simulink model "car_model_FIXED"  (R2022b)
settings: Solver=VariableStepAuto  StartTime=0.0  StopTime=60  RelTol=1e-3
values from neighbouring files (symbols this model uses):
  ABS_MAX_TORQUE = [25 25 25 25]    [workspace.mat]
  ABS_MAX_TRQ_CMD = 50    [workspace.mat]
  ABS_MIN_TORQUE = [0.01 0.01 0.01 0.01]    [workspace.mat]
  acc_IC = 0    [workspace.mat]
  ACCELERATION_MAX = 30    [workspace.mat]
  ActSuspDutyCycle = 1    [workspace.mat]
  Aeq_left = [0.305756190204 0.308857786592 0.311945941182 0.315020811431 0.318082554689 0.321131328186 0.324167289011 0.327190594103 0.330201400225 0.333199863958 0.336186141681 0.339160389558 ... (261 elements, 1x261)]    [workspace.mat]
  Aeq_right = [-0.961664782545 -0.959835898365 -0.957982924115 -0.956106413788 -0.954206913862 -0.952284963337 -0.950341093764 -0.948375829284 -0.946389686656 -0.944383175301 -0.942356797333 -0.940311047601 ... (261 elements, 1x261)]    [workspace.mat]
  alpha_error = 0.1    [workspace.mat]
  ang_acc_hystersesis = 0.1    [workspace.mat]
  ang_IC = 0    [workspace.mat]
  ang_vel_IC = 0    [workspace.mat]
  area_air = 0.15    [workspace.mat]
  axb = -5    [workspace.mat]
  battery_current_IC = 0    [workspace.mat]
  BATTERY_CURRENT_MAX = 140    [workspace.mat]
  BATTERY_CURRENT_MIN = 0    [workspace.mat]
  battery_FT_IC = 300    [workspace.mat]
  battery_T_IC = 300    [workspace.mat]
  BATTERY_TEMPERATURE_MAX = 60    [workspace.mat]
  BATTERY_TEMPERATURE_MIN = 0    [workspace.mat]
  battery_voltage_IC = 332    [workspace.mat]
  BATTERY_VOLTAGE_MAX = 340    [workspace.mat]
  BATTERY_VOLTAGE_MIN = 60    [workspace.mat]
  br = 0.01    [workspace.mat]
  brake_bias = [0.35 0.35 0.15 0.15]    [workspace.mat]
  Brake_Pressure_IC = 1    [workspace.mat]
  ccl_IC = 0    [workspace.mat]
  CENTER_STEER_ANGLE_MAX = 130    [workspace.mat]
  covarience_matrix_IC = [0.001 0 0 0 0 0 0 0 0 0 0 0 ... (784 elements, 28x28)]    [workspace.mat]
  CURRENT_BUFFER = 25    [workspace.mat]
  cy_sweep = [13568.4166816 14020.2069783 14456.754831 14879.7402576 15289.7264712 15687.2766846 16072.954111 16447.3219632 16810.9434544 17164.3817975 17508.2002054 17842.9618912 ... (101 elements, 1x101)]    [workspace.mat]
  dB = 0.001    [workspace.mat]
  dcl_IC = 140    [workspace.mat]
  DCL_MAX = 130    [workspace.mat]
  DCL_MIN = 0    [workspace.mat]
  deadband_angle = 12    [workspace.mat]
  dIndex = 50    [workspace.mat]
  driver_t = 0.015    [workspace.mat]
  dt_OFF = 4.5    [workspace.mat]
  dt_ON = 7.5    [workspace.mat]
  dTx = 0.01    [workspace.mat]
  dx = 0.1    [workspace.mat]
  dZ = 0.295    [workspace.mat]
  efficiency_grid = [0.759500051293 0.787587791453 0.809832189108 0.826747821898 0.837164543102 0.842744381136 0.842258400104 0.838611650621 0.82826195101 0.814029316176 0.795690627225 0.7759791486 ... (2782 elements, 26x107)]    [workspace.mat]
  F0z = [0 0]    [workspace.mat]
  forward_look_straight = 5    [workspace.mat]
  forward_look_turn = 15    [workspace.mat]
  Fz_IC = 539.55    [workspace.mat]
  Fz_sweep = [200 210 220 230 240 250 260 270 280 290 300 310 ... (101 elements, 1x101)]    [workspace.mat]
  g = 9.81    [workspace.mat]
  GAIN_ABS = 100    [workspace.mat]
  gearbox_efficiency = [0.8 0.8 0.8 0.8]    [workspace.mat]
  gps_counter_IC = 0    [workspace.mat]
  gps_hz = 0.01    [workspace.mat]
  gr = [8.74786324786 8.74786324786 8.74786324786 8.74786324786]    [workspace.mat]
  I = 0    [workspace.mat]
  I_Driver = 1    [workspace.mat]
  indicies = [3 3.5 4 0.5 1 1.5 2 2.5 3 3.5 4 0.5 ... (27 elements, 1x27)]    [workspace.mat]
  IYY = 0.3    [workspace.mat]
  kx_sweep = [8779.958 9178.302 9576.646 9974.99 10373.334 10771.678 11170.022 11568.366 11966.71 12365.054 12763.398 13161.742 ... (101 elements, 1x101)]    [workspace.mat]
  l = [0.772 0.772]    [workspace.mat]
  lambda_star = 0.15    [workspace.mat]
  low_V_SA = 0.001    [workspace.mat]
  lr = 35    [workspace.mat]
  m_all = 220    [workspace.mat]
  m_body = 180    [workspace.mat]
  m_unsprung = [6 6 14 14]    [workspace.mat]
  MAG_MAX = 200    [workspace.mat]
  Max_Brake_Pressure = 100000000    [workspace.mat]
  Max_Driver_Input = 1    [workspace.mat]
  MAX_DTHETA_DRIVER = 360    [workspace.mat]
  MAX_I_Driver = 1    [workspace.mat]
  MAX_STEERING_ADJUST = 15    [workspace.mat]
  max_yaw = [0.705271610162 0.928228152446 1.12280857731 1.14131008363 1.08727026041 1.01377803859 0.938114723816 0.8718206875 0.815009168116 0.767481919497 0.727119764215 0.694403589394 ... (15 elements, 1x15)]    [workspace.mat]
  Min_Brake_Pressure = 1    [workspace.mat]
  Min_Driver_Input = 0    [workspace.mat]
  min_velocity_regen = 1.4    [workspace.mat]
  motor_current_IC = 0    [workspace.mat]
  MOTOR_CURRENT_MAX = 70    [workspace.mat]
  MOTOR_CURRENT_MIN = 0    [workspace.mat]
  MOTOR_ENABLE = [0 0 1 1]    [workspace.mat]
  motor_FT_IC = 300    [workspace.mat]
  motor_T_IC = 300    [workspace.mat]
  MOTOR_TEMPERATURE_MAX = 100    [workspace.mat]
  MOTOR_TEMPERATURE_MIN = 0    [workspace.mat]
  motor_voltage_IC = 332    [workspace.mat]
  MOTOR_VOLTAGE_MAX = 340    [workspace.mat]
  MOTOR_VOLTAGE_MIN = 90    [workspace.mat]
  motorControllerCurve = [25  260; 50  130; 75  0]    [workspace.mat]
  motorTempCurve = [140 138.6 134.4 127.4 117.6 105 89.6 71.4 50.4 26.6 0]    [workspace.mat]
  motorTempX = [75 77 79 81 83 85 87 89 91 93 95]    [workspace.mat]
  mu_star = 0.5    [workspace.mat]
  mx_sweep = [3.38348 3.3655067 3.3477908 3.3303323 3.3131312 3.2961875 3.2795012 3.2630723 3.2469008 3.2309867 3.21533 3.1999307 ... (101 elements, 1x101)]    [workspace.mat]
  my_sweep = [3.036232 3.015241699 2.994987032 2.975452753 2.956623616 2.938484375 2.921019784 2.904214597 2.888053568 2.872521451 2.857603 2.843282969 ... (101 elements, 1x101)]    [workspace.mat]
  noise_state = [1e-06 1e-06 1e-06 1e-06 0.005 0.005 0.005 1e-06 1e-06 1e-06 1e-06 1e-06 ... (28 elements, 28x1)]    [workspace.mat]
  omega_IC = 0    [workspace.mat]
  OMEGA_MAX = 150    [workspace.mat]
  OMEGA_MIN = 0    [workspace.mat]
  ORIENTATION_MAX = 360    [workspace.mat]
  P = 2    [workspace.mat]
  P_Driver = 0.7    [workspace.mat]
  P_High_Speed = 0.1    [workspace.mat]
  P_Steering_Adjust = 2    [workspace.mat]
  P_Straight_Adjust = 5    [workspace.mat]
  pos_IC = 0    [workspace.mat]
  POS_MAX = 300    [workspace.mat]
  q_thresh = 0.3    [workspace.mat]
  RE = 0.223    [workspace.mat]
  rho = 1.225    [workspace.mat]
  s = [0.649 0.621]    [workspace.mat]
  selected_maxvm = [49.86390724 16.21289794 8.219813569 8.05215527 7.103352929 8.35634983 13.87515039 8.72402841 22.75224945 36.67909339 19.32001297 25.09036962 ... (63 elements, 21x3)]    [workspace.mat]
  selected_sweep = [3 3 3 3 3 3 3 3 3 3 3 3 ... (1288 elements, 644x2)]    [workspace.mat]
  selected_track = [inf inf inf inf inf inf inf inf inf inf inf inf ... (37971 elements, 4219x9)]    [workspace.mat]
  shock_length_IC = 0.1    [workspace.mat]
  SHOCK_LENGTH_MAX = 0.25    [workspace.mat]
  SHOCK_LENGTH_MIN = 0    [workspace.mat]
  state_IC = [1 0 0 0 0 0 0 0 0 0 0 0 ... (28 elements, 28x1)]    [workspace.mat]
  steering_sweep = [0 5 10 15 20 25 30 35 40 45 50 55 ... (27 elements, 1x27)]    [workspace.mat]
  steering_Up_Grid = [0.551231966244 8.36038106007 16.1333806643 23.9559539118 31.8240691982 39.7561724339 47.7157531433 55.7845698794 64.1341708168 73.0798046026 82.7903081349 93.1297322155 ... (615 elements, 41x15)]    [workspace.mat]
  ... (+25 more)
undefined symbols (not defined in the file or in its folder): ax, ay, az, covA, covG, covM, covP, covV, DiscIntNeverNeededParam, fusion_t, fusion_t_sim, gps_ratio, IMU_accel, IMU_gyro, imu_hz, IMU_mag, location_lla_IC, p, phi, psi, q, r, sus, theta, trn, veh, VEH, whl, X, Xdot, Y, Ydot, Z, Zdot
libraries: fl_lib x82, nesl_utility x32, vehdynlibtire x10, vehdynlibsuspension x8, simulink x5, autolibutils x5, sharedtransform x5, sdl_lib x4, EngineCoolingComponents_lib x4, slpidlib x3, SimscapeFluids_lib x3, shared6dof x2
(part 3 of 14)

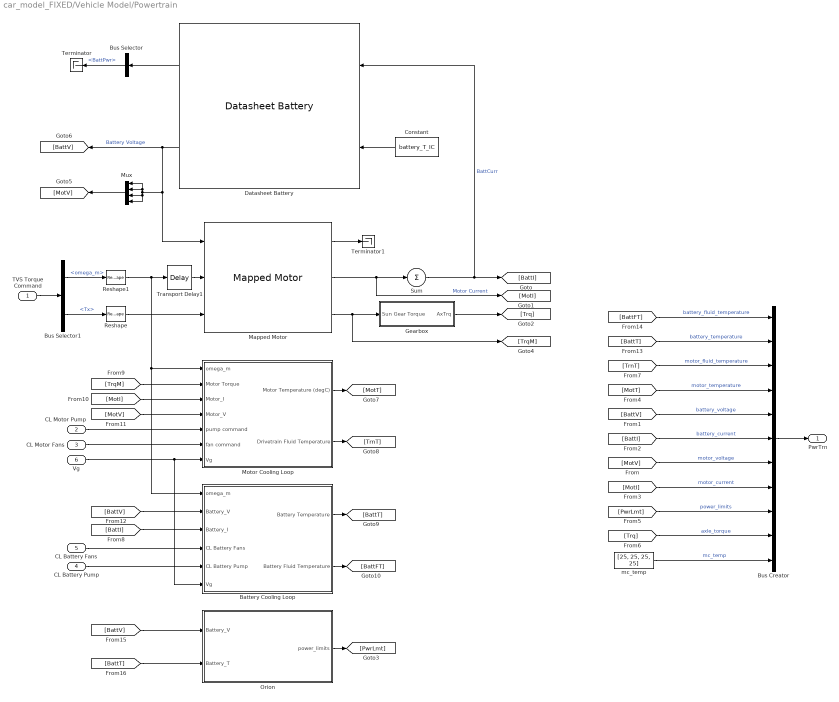
== system car_model_FIXED/Vehicle Model/Powertrain ==
  TVS Torque Command : Inport
  CL Motor Pump : Inport  Port=2
  CL Motor Fans : Inport  Port=3
  CL Battery Pump : Inport  Port=4
  CL Battery Fans : Inport  Port=5
  Vg : Inport  Port=6
  Battery Cooling Loop : Subsystem
  Bus Creator : BusCreator  Inputs=11
  Bus Selector : BusSelector  OutputSignals=BattPwr
  Bus Selector1 : BusSelector  OutputSignals=omega_m,Tx
  Constant : Constant  Value=battery_T_IC
  Datasheet Battery : autolibdatasheetbattery/Datasheet Battery  CapacityCtrl=Parameter  OutputVlt=Filtered  BattChargeMax=BattCap  Em=Em  CapLUTBp=SOC  RInt=RESISTANCE  BattTempBp=TEMPERATURE  CapSOCBp=SOC  Ns=Ns  Np=Np  BattCapInit=BattCap_I  Tc=Battery_tau  Vinit=battery_voltage_IC  RefBlkName='autolibdatasheetbattery/Datasheet Battery'
  Gearbox : Subsystem
  Mapped Motor : autolibmappedmotor/Mapped Motor  port_config=Speed  param_by=Tabulated torque-speed envelope  w_t=rpm_sweep  T_t=max_torque_grid(end,:)  torque_max=.1  power_max=30  Tc=Motor_tau  param_loss=Tabulated efficiency data  eff=100  w_eff=375  T_eff=0.08  Piron=0  Pbase=0  w_eff_bp=rpm_sweep  T_eff_bp=torque_sweep  Temp_eff_bp=[233.15 293.15 373.15]  losses_table=[1.49 1.67 2.21 3.10; 0.42 0.69 1.14 2.03; 0.06 0.24 0.78 1.68; 0.42 0.69 1.14 2.03; 1.49 1.67 2.21 3.10]  losses_table_3d=cat(3,[1.49 1.67 2.21 3.10; 0.42 0.69 1.14 2.03; 0.06 0.24 0.78 1.68; 0.42 0.69 1.14 2.03; 1.49 1.67 2.21 3.10],[1.49 1.67 2.21 3.10; 0.42 0.69 1.14 2.03; 0.06 0.24 0.78 1.68; 0.42 0.69 1.14 2.03; 1.49 1.67 2.21 3.10],[1.49 1.67 2.21 3.10; 0.42 0.69 1.14 2.03; 0.06 0.24 0.78 1.68; 0.42 0.69 1.14 2.03; 1.49 1.67 2.21 3.10])  efficiency_table=100*efficiency_grid'  efficiency_table_3d=cat(3,[95 95 95 95; 95 95 95 95; 95 95 95 95; 95 95 95 95; 95 95 95 95],[95 95 95 95; 95 95 95 95; 95 95 95 95; 95 95 95 95; 95 95 95 95],[95 95 95 95; 95 95 95 95; 95 95 95 95; 95 95 95 95; 95 95 95 95])  J=5e-6  b=1e-5  omega_o=0  T_t_extended=[1.32786372122435 1.93296548257099 2.5425618526431 3.15736795662177 3.77818881981173 4.40971488438617 5.05604488344693 5.69719862521611 6.35896558084689 7.05699514881516 7.75957227021141 8.48856911751552 9.2939724316526 10.1031648805232 10.9920408781878 11.9746245835295 13.0147067052248 14.1174245714548 15.288285754278 16.5327710759749 17.9226945866055 19.3096243918455 20.7636741817153 22.2031334917467 23.663316115528 25 25 25 25 25 25 25 25 25 25 25 25 25 25 25 25 25 25 25 25 25 25 25 25 25 25 25 25 25 25 25 25 25 25 25 25 25 25 25 25 25 25 25 25 25 25 25 25 25 25 25 25 25 25 25 25 25 25 25 25 25 25 25 25 25 25 25 25 25 25 25 25 25 25 25 25 25 25 25 25 25 25 25 25 25 25 25 25 25 25 25 25 25 25 25 25 25 25 25 25 25 25 25 25 25 25 25 25 25 25 25 25 25 25 25 25 25 25 25 25 25 25 25 25 25 25 25 25 25 25 25 25 25 25 25 25 25 25 25 25 25 25 25 25 25 25 25 25 25 25 25 25 25 25 25 25 25 25 25 25 25 25 25 23.663316115528 22.2031334917467 20.7636741817153 19.3096243918455 17.9226945866055 16.5327710759749 15.288285754278 14.1174245714548 13.0147067052248 11.9746245835295 10.9920408781878 10.1031648805232 9.2939724316526 8.48856911751552 7.75957227021141 7.05699514881516 6.35896558084689 5.69719862521611 5.05604488344693 4.40971488438617 3.77818881981173 3.15736795662177 2.5425618526431 1.93296548257099 1.32786372122435]  w_t_extended=[-1100 -1089.62264150943 -1079.24528301887 -1068.8679245283 -1058.49056603774 -1048.11320754717 -1037.7358490566 -1027.35849056604 -1016.98113207547 -1006.60377358491 -996.22641509434 -985.849056603774 -975.471698113208 -965.094339622642 -954.716981132075 -944.339622641509 -933.962264150943 -923.584905660377 -913.207547169811 -902.830188679245 -892.452830188679 -882.075471698113 -871.698113207547 -861.320754716981 -850.943396226415 -840.566037735849 -830.188679245283 -819.811320754717 -809.433962264151 -799.056603773585 -788.679245283019 -778.301886792453 -767.924528301887 -757.547169811321 -747.169811320755 -736.792452830189 -726.415094339623 -716.037735849057 -705.660377358491 -695.283018867925 -684.905660377358 -674.528301886792 -664.150943396226 -653.77358490566 -643.396226415094 -633.018867924528 -622.641509433962 -612.264150943396 -601.88679245283 -591.509433962264 -581.132075471698 -570.754716981132 -560.377358490566 -550 -539.622641509434 -529.245283018868 -518.867924528302 -508.490566037736 -498.11320754717 -487.735849056604 -477.358490566038 -466.981132075472 -456.603773584906 -446.22641509434 -435.849056603774 -425.471698113208 -415.094339622641 -404.716981132075 -394.339622641509 -383.962264150943 -373.584905660377 -363.207547169811 -352.830188679245 -342.452830188679 -332.075471698113 -321.698113207547 -311.320754716981 -300.943396226415 -290.566037735849 -280.188679245283 -269.811320754717 -259.433962264151 -249.056603773585 -238.679245283019 -228.301886792453 -217.924528301887 -207.547169811321 -197.169811320755 -186.792452830189 -176.415094339623 -166.037735849057 -155.660377358491 -145.283018867925 -134.905660377358 -124.528301886792 -114.150943396226 -103.77358490566 -93.3962264150943 -83.0188679245283 -72.6415094339623 -62.2641509433962 -51.8867924528302 -41.5094339622642 -31.1320754716981 -20.7547169811321 -10.377358490566 0 10.377358490566 20.7547169811321 31.1320754716981 41.5094339622642 51.8867924528302 62.2641509433962 72.6415094339623 83.0188679245283 93.3962264150943 103.77358490566 114.150943396226 124.528301886792 134.905660377358 145.283018867925 155.660377358491 166.037735849057 176.415094339623 186.792452830189 197.169811320755 207.547169811321 217.924528301887 228.301886792453 238.679245283019 249.056603773585 259.433962264151 269.811320754717 280.188679245283 290.566037735849 300.943396226415 311.320754716981 321.698113207547 332.075471698113 342.452830188679 352.830188679245 363.207547169811 373.584905660377 383.962264150943 394.339622641509 404.716981132075 415.094339622641 425.471698113208 435.849056603774 446.22641509434 456.603773584906 466.981132075472 477.358490566038 487.735849056604 498.11320754717 508.490566037736 518.867924528302 529.245283018868 539.622641509434 550 560.377358490566 570.754716981132 581.132075471698 591.509433962264 601.88679245283 612.264150943396 622.641509433962 633.018867924528 643.396226415094 653.77358490566 664.150943396226 674.528301886792 684.905660377358 695.283018867925 705.660377358491 716.037735849057 726.415094339623 736.792452830189 747.169811320755 757.547169811321 767.924528301887 778.301886792453 788.679245283019 799.056603773585 809.433962264151 819.811320754717 830.188679245283 840.566037735849 850.943396226415 861.320754716981 871.698113207547 882.075471698113 892.452830188679 902.830188679245 913.207547169811 923.584905660377 933.962264150943 944.339622641509 954.716981132075 965.094339622642 975.471698113208 985.849056603774 996.22641509434 1006.60377358491 1016.98113207547 1027.35849056604 1037.7358490566 1048.11320754717 1058.49056603774 1068.8679245283 1079.24528301887 1089.62264150943 1100]  KLossIron=0  KLossCopper=0  x_w_eff_vec=[-1100 -1089.62264150943 -1079.24528301887 -1068.8679245283 -1058.49056603774 -1048.11320754717 -1037.7358490566 -1027.35849056604 -1016.98113207547 -1006.60377358491 -996.22641509434 -985.849056603774 -975.471698113208 -965.094339622642 -954.716981132075 -944.339622641509 -933.962264150943 -923.584905660377 -913.207547169811 -902.830188679245 -892.452830188679 -882.075471698113 -871.698113207547 -861.320754716981 -850.943396226415 -840.566037735849 -830.188679245283 -819.811320754717 -809.433962264151 -799.056603773585 -788.679245283019 -778.301886792453 -767.924528301887 -757.547169811321 -747.169811320755 -736.792452830189 -726.415094339623 -716.037735849057 -705.660377358491 -695.283018867925 -684.905660377358 -674.528301886792 -664.150943396226 -653.77358490566 -643.396226415094 -633.018867924528 -622.641509433962 -612.264150943396 -601.88679245283 -591.509433962264 -581.132075471698 -570.754716981132 -560.377358490566 -550 -539.622641509434 -529.245283018868 -518.867924528302 -508.490566037736 -498.11320754717 -487.735849056604 -477.358490566038 -466.981132075472 -456.603773584906 -446.22641509434 -435.849056603774 -425.471698113208 -415.094339622641 -404.716981132075 -394.339622641509 -383.962264150943 -373.584905660377 -363.207547169811 -352.830188679245 -342.452830188679 -332.075471698113 -321.698113207547 -311.320754716981 -300.943396226415 -290.566037735849 -280.188679245283 -269.811320754717 -259.433962264151 -249.056603773585 -238.679245283019 -228.301886792453 -217.924528301887 -207.547169811321 -197.169811320755 -186.792452830189 -176.415094339623 -166.037735849057 -155.660377358491 -145.283018867925 -134.905660377358 -124.528301886792 -114.150943396226 -103.77358490566 -93.3962264150943 -83.0188679245283 -72.6415094339623 -62.2641509433962 -51.8867924528302 -41.5094339622642 -31.1320754716981 -20.7547169811321 -10.377358490566 0 10.377358490566 20.7547169811321 31.1320754716981 41.5094339622642 51.8867924528302 62.2641509433962 72.6415094339623 83.0188679245283 93.3962264150943 103.77358490566 114.150943396226 124.528301886792 134.905660377358 145.283018867925 155.660377358491 166.037735849057 176.415094339623 186.792452830189 197.169811320755 207.547169811321 217.924528301887 228.301886792453 238.679245283019 249.056603773585 259.433962264151 269.811320754717 280.188679245283 290.566037735849 300.943396226415 311.320754716981 321.698113207547 332.075471698113 342.452830188679 352.830188679245 363.207547169811 373.584905660377 383.962264150943 394.339622641509 404.716981132075 415.094339622641 425.471698113208 435.849056603774 446.22641509434 456.603773584906 466.981132075472 477.358490566038 487.735849056604 498.11320754717 508.490566037736 518.867924528302 529.245283018868 539.622641509434 550 560.377358490566 570.754716981132 581.132075471698 591.509433962264 601.88679245283 612.264150943396 622.641509433962 633.018867924528 643.396226415094 653.77358490566 664.150943396226 674.528301886792 684.905660377358 695.283018867925 705.660377358491 716.037735849057 726.415094339623 736.792452830189 747.169811320755 757.547169811321 767.924528301887 778.301886792453 788.679245283019 799.056603773585 809.433962264151 819.811320754717 830.188679245283 840.566037735849 850.943396226415 861.320754716981 871.698113207547 882.075471698113 892.452830188679 902.830188679245 913.207547169811 923.584905660377 933.962264150943 944.339622641509 954.716981132075 965.094339622642 975.471698113208 985.849056603774 996.22641509434 1006.60377358491 1016.98113207547 1027.35849056604 1037.7358490566 1048.11320754717 1058.49056603774 1068.8679245283 1079.24528301887 1089.62264150943 1100]  x_T_eff_vec=[-25 -24 -23 -22 -21 -20 -19 -18 -17 -16 -15 -14 -13 -12 -11 -10 -9 -8 -7 -6 -5 -4 -3 -2 -1 0 1 2 3 4 5 6 7 8 9 10 11 12 13 14 15 16 17 18 19 20 21 22 23 24 25]  x_tmp_eff_vec=[-0.09 -0.06 -0.03 0 0.03 0.06 0.09]  x_losses_mat=[23585.2454984914 25575.6048947257 27139.4520082014 29267.8482790089 31020.3464218685 31596.6371464587 31518.9940065617 29885.8513636213 26591.5997195433 22791.5674419838 18877.9321448778 15399.2342103956 12463.5759285319 10150.4360770642 7940.12577685447 5941.78114713604 4281.75749355199 3087.40993350763 2320.6792119085 1832.65329562565 1523.89345075454 1324.52413374058 1161.36806266051 963.589049891181 633.00086054754 0 401.789152246756 670.092061999493 859.044703990233 1018.05950194334 1193.27179973802 1434.36606808011 1783.23540289163 2285.5447542264 2989.00888732852 3857.89381003457 4794.15763003356 5738.04085607008 6659.39171409456 7699.80854783878 8804.52478440242 9931.07255753513 10979.1422213972 11909.6249889955 12566.951869673 12969.5826871112 13240.307014288 13246.8754803077 13093.7320950667 12990.6322511943 12696.3127000665;20656.2459033155 21993.4435343943 23437.7073112699 24870.7678351695 25278.6164625767 26544.2281776888 25364.6741409987 23823.6941510163 21803.0981873599 18639.918112837 15570.0939757232 12757.0747130636 10521.1777863946 8506.09888485944 6779.07461503079 5240.82738593529 3821.40652629411 2768.00706527213 2102.14227188113 1678.08902010339 1419.31391863137 1251.68707752293 1111.01448170121 931.394117223434 616.881829183563 0 393.886110325397 652.514153981521 829.191121148383 972.423097025598 1125.97960832735 1335.33795076621 1647.95636459537 2100.8872579426 2749.85260772004 3538.76503751473 4330.04506178925 5153.52924861191 6037.09928933147 6947.27300486337 7973.91259071895 9008.39126786498 10014.9952712058 10757.191228114 11398.9361736269 11967.3885011214 12010.359205515 12206.4790712756 12111.1684935981 11946.3416947208 11747.9182396002;18278.8851920739 19412.0163288424 20382.1425992281 21165.0085600588 21585.0313058547 22053.3159769321 21161.8127388475 19985.0892819494 18131.9686198184 15504.1953878283 12966.5407209478 10731.1550972048 8929.32297354866 7255.70507255164 5819.24119948282 4575.57400567279 3382.28418096587 2487.86784339288 1912.55742024297 1545.13237368107 1326.24931789792 1184.94225865936 1065.00386922092 901.593411675841 601.979911728552 0 386.434834687782 635.956688665174 801.396652489346 929.742748117063 1064.59909808497 1247.46974991523 1526.18688415761 1931.3509440752 2508.71283914039 3213.27306066569 3905.06538670013 4650.36177768533 5456.56580119647 6274.68974901775 7199.77996720502 8169.29989619905 9119.46722396751 9850.89623531754 10414.2851135192 10908.2984365612 11055.7163492463 11190.092072215 11192.1476655798 11096.1054936499 10896.704096341;16356.191001019 17008.7874387829 17716.4948506901 18136.1341764628 18754.2009913978 18310.9705064106 17970.2318327614 16730.1580570695 15114.1837198323 12930.9675590827 10921.7678045366 9152.91727398149 7630.24575997576 6198.4633808774 5014.66917186725 3976.08010013008 2985.3111047389 2219.07242333604 1738.73788172918 1427.459222716 1242.23863816208 1124.85815589397 1022.88435631936 874.310512232978 588.221715288471 0 379.419018063734 620.523292479225 775.503970261498 890.556565974922 1007.95054910588 1167.57828499485 1410.86990463404 1761.8509575081 2278.29041178213 2898.03902285899 3515.34991727439 4178.95254226008 4925.5200849043 5679.19924701238 6496.39380971728 7363.40078514735 8251.06303386496 8948.67640278782 9533.97242057888 9862.85365794915 10217.3950171393 10239.1435093175 10296.3814239629 10227.5431675514 10145.9288558048;14455.6070797839 14902.5902769716 15562.2431472041 15880.8692382896 16080.5414854643 15608.1598281898 15310.6638060815 14261.9872763884 12693.0914336588 10951.0155073205 9325.25473251517 7886.08989012305 6529.93490084548 5365.39558685114 4344.80491672476 3475.14714022565 2662.76511687903 2009.70096597575 1583.99145564077 1320.41659976618 1165.70696024761 1070.18501668943 984.100718072373 849.23019374686 575.801237442044 0 372.932285683337 606.094475231797 751.275291222694 854.260399723461 955.29520809771 1093.14268772857 1305.00666231077 1624.22259830077 2081.0756230161 2616.21383339621 ...(+175555 chars)]  x_losses_mat_3d=[37.8947368421052 25.2631578947368 12.6315789473684 0 12 24 36;18.9473684210526 12.6315789473684 6.3157894736842 0 5.99999999999999 12 18;0 0 0 0 0 0 0;18 12 5.99999999999999 0 6.3157894736842 12.6315789473684 18.9473684210526;36 24 12 0 12.6315789473684 25.2631578947368 37.8947368421052]  CalLossMapData={}  CalLossWithTempMapData={}  aMode=1  RefBlkName='autolibmappedmotor/Mapped Motor'
  Motor Cooling Loop : Subsystem
  Mux : Mux
  Orion : Subsystem
  Reshape : Reshape  OutputDimensionality=Customize  OutputDimensions=[1,4]
  Reshape1 : Reshape  OutputDimensionality=Customize  OutputDimensions=[1,4]
  Sum : Sum  Inputs=+
  Terminator : Terminator
  Terminator1 : Terminator
  Transport Delay1 : TransportDelay  DelayTime=0.001  InitialOutput=omega_IC
  mc_temp : Constant  Value=[25, 25, 25, 25]
  PwrTrn : Outport
  wires:
  [BattT] -> Orion/2(Battery_T)
  [Trq] -> Bus Creator/10  "axle_torque"
  [TrnT] -> Bus Creator/3  "motor_fluid_temperature"
  Vg/1 -> Motor Cooling Loop/7(Vg), Battery Cooling Loop/6(Vg)
  CL Battery Fans/1 -> Battery Cooling Loop/4(CL Battery Fans)
  [MotT] -> Bus Creator/4  "motor_temperature"
  Battery Cooling Loop/2(Battery Fluid Temperature) -> [BattFT]
  [BattI] -> Bus Creator/6  "battery_current"
  [MotI] -> Bus Creator/8  "motor_current"
  [MotV] -> Motor Cooling Loop/4(Motor_V)
  Motor Cooling Loop/2(Drivetrain Fluid Temperature) -> [TrnT]
  Mux/1 -> [MotV]
  CL Battery Pump/1 -> Battery Cooling Loop/5(CL Battery Pump)
  Mapped Motor/1 -> Terminator1/1
  Bus Selector1/1 -> Reshape1/1  "<omega_m>"
  Transport Delay1/1 -> Mapped Motor/2
  Bus Selector1/2 -> Reshape/1  "<Tx>"
  CL Motor Pump/1 -> Motor Cooling Loop/5(pump command)
  Battery Cooling Loop/1(Battery Temperature) -> [BattT]
  Sum/1 -> [BattI], Datasheet Battery/1  "BattCurr"
  Datasheet Battery/1 -> Bus Selector/1
  [BattI] -> Battery Cooling Loop/3(Battery_I)
  [BattV] -> Orion/1(Battery_V)
  Bus Selector/1 -> Terminator/1  "<BattPwr>"
  Motor Cooling Loop/1(Motor Temperature (degC)) -> [MotT]
  Datasheet Battery/2 -> [BattV], Mux/1, Mux/2, Mux/4, Mux/3, Mapped Motor/1  "Battery Voltage"
  [MotV] -> Bus Creator/7  "motor_voltage"
  [BattV] -> Bus Creator/5  "battery_voltage"
  [MotI] -> Motor Cooling Loop/3(Motor_I)
  [BattV] -> Battery Cooling Loop/2(Battery_V)
  [BattFT] -> Bus Creator/1  "battery_fluid_temperature"
  Mapped Motor/2 -> Sum/1, [MotI]  "Motor Current"
  Constant/1 -> Datasheet Battery/2
  Bus Creator/1 -> PwrTrn/1
  CL Motor Fans/1 -> Motor Cooling Loop/6(fan command)
  [PwrLmt] -> Bus Creator/9  "power_limits"
  [BattT] -> Bus Creator/2  "battery_temperature"
  Orion/1(power_limits) -> [PwrLmt]
  [TrqM] -> Motor Cooling Loop/2(Motor Torque)
  Gearbox/1(AxTrq) -> [Trq]
  mc_temp/1 -> Bus Creator/11  "mc_temp"
  Reshape/1 -> Mapped Motor/3
  Reshape1/1 -> Motor Cooling Loop/1(omega_m), Battery Cooling Loop/1(omega_m), Transport Delay1/1
  Mapped Motor/3 -> Gearbox/1(Sun Gear Torque), [TrqM]
  TVS Torque Command/1 -> Bus Selector1/1
